simulink library "GRC_Lib"  (R2017b)
settings: Solver=VariableStepAuto  StartTime=0.0  StopTime=10.0  RelTol=1e-3  EnableMultiTasking=on
StartFcn:
  | set_param('AdvancedOperations','ZoomFactor','100');
undefined symbols (not defined in the file): Test
libraries: GRC_Lib x203, simulink x1
(part 2 of 4)

== system GRC_Lib/Constants_Parameters ==
  note: // 1D/2D Lookup Table just allow
      | -- 'double' input data type
      | -- 'Linear' Lookup method
  CalConstant : Subsystem  mask{slddName=CalParam.sldd, CalParamNameMsk=Test, IniVal=0, CPDT=double, MinVal=0, MaxVal=10, StrgClss=SimulinkGlobal}
      mask prompts: slddName "Linked sldd Name"; CalParamNameMsk "Calibration Parameter Name"; IniVal "Initial Value"; CPDT "Calibration Parameter Data Type"; MinVal "Min Value"; MaxVal "Max Value"; StrgClss "Storage Class"
      mask init:
      | CalParamName = CalParamNameMsk;
      | ParamVal = IniVal;
      | ParamMin = MinVal;
      | ParamMax = MaxVal;
      | 
      | set_param(gcb,'slddName',get_param(gcs,'DataDictionary'));
      | % slddName = get_param(gcs,'DataDictionary')
      | 
      | Caldd = Simulink.data.dictionary.open(get_param(gcs,'DataDictionary'));  
      | clc;
      | if ~exist(getSection(Caldd,'Design Data'),get_param(gcb,'CalParamNameMsk'))
      |     importFromFile(getSection(Caldd,'Design Data'),'CalParamDef.m');
      | else
      |     warning('*** The parameter %s has added to sldd, please confirm ***',get_param(gcb,'CalParamNameMsk'));
      | end
      | 
      | try
      | if exist(getSection(Caldd,'Design Data'),'Test')
      |     deleteEntry(getEntry(getSection(Simulink.data.dictionary.open(get_param(gcs,'DataDictionary')),'Design Data'),'Test'));
      | else
      | end
      | catch
      | end
      | 
      | saveChanges(Caldd);
      | fprintf('%s save finished.\n',get_param(gcb,'slddName')); 
      | clear;
      | 
      | DTStry = get_param(gcb,'CPDT');
      | try
      |     if isequal(DTStry,'boolean')
      |         FColor = '[0.901961, 0.313725, 0.078431]'; 
      |     elseif isequal(DTStry,'double')||isequal(DTStry,'single')
      |         FColor = '[0.313725, 0.117647, 0.352941]';  
      |     else
      |         FColor = '[0.196078, 0.549020, 0.549020]';
      |     end        
      | catch
      | end
      | set_param([gcb '/Out'],'ForegroundColor',FColor);
      | set_param(gcb,'ForegroundColor',FColor);
      settings: AttributesFormatString=%<slddName>
      mask Callback CalParamNameMsk:
      | FileFullPath = which(get_param(gcs,'DataDictionary'));
      | [ParentPathStr,name,ext] = fileparts(FileFullPath);
      | cd(ParentPathStr);
      | 
      | if ~exist(getSection(Simulink.data.dictionary.open(get_param(gcs,'DataDictionary')),'Design Data'),get_param(gcb,'CalParamNameMsk'))
      | %    try
      |    fid = fopen('CalParamDef.m','w');
      |    fprintf(fid,'%s',strcat(get_param(gcb,'CalParamNameMsk'),' = Simulink.Parameter;'));
      |    fprintf(fid,'\r');
      |    fprintf(fid,'%s',strcat(get_param(gcb,'CalParamNameMsk'),'.Value = ',get_param(gcb,'IniVal'),';'));
      |    fprintf(fid,'\r');
      |    fprintf(fid,'%s',strcat(get_param(gcb,'CalParamNameMsk'),'.Min = ',get_param(gcb,'MinVal'),';'));
      |    fprintf(fid,'\r');
      |    fprintf(fid,'%s',strcat(get_param(gcb,'CalParamNameMsk'),'.Max = ',get_param(gcb,'MaxVal'),';'));
      |    fprintf(fid,'\r');
      |    fprintf(fid,'%s',strcat(get_param(gcb,'CalParamNameMsk'),'.DataType = ','''', get_param(gcb,'CPDT')),'''',';');
      |    fprintf(fid,'\r');
      |    fprintf(fid,'%s',strcat(get_param(gcb,'CalParamNameMsk'),'.StorageClass = ','''',get_param(gcb,'StrgClss')),'''',';');
      |    fclose(fid);
      | %    catch
      | %    end
      | clear;
      | clc;
      | else
      | end
      mask Callback IniVal:
      | FileFullPath = which(get_param(gcs,'DataDictionary'));
      | [ParentPathStr,name,ext] = fileparts(FileFullPath);
      | cd(ParentPathStr);
      | 
      | if ~exist(getSection(Simulink.data.dictionary.open(get_param(gcs,'DataDictionary')),'Design Data'),get_param(gcb,'CalParamNameMsk'))
      | %    try
      |    fid = fopen('CalParamDef.m','w');
      |    fprintf(fid,'%s',strcat(get_param(gcb,'CalParamNameMsk'),' = Simulink.Parameter;'));
      |    fprintf(fid,'\r');
      |    fprintf(fid,'%s',strcat(get_param(gcb,'CalParamNameMsk'),'.Value = ',get_param(gcb,'IniVal'),';'));
      |    fprintf(fid,'\r');
      |    fprintf(fid,'%s',strcat(get_param(gcb,'CalParamNameMsk'),'.Min = ',get_param(gcb,'MinVal'),';'));
      |    fprintf(fid,'\r');
      |    fprintf(fid,'%s',strcat(get_param(gcb,'CalParamNameMsk'),'.Max = ',get_param(gcb,'MaxVal'),';'));
      |    fprintf(fid,'\r');
      |    fprintf(fid,'%s',strcat(get_param(gcb,'CalParamNameMsk'),'.DataType = ','''', get_param(gcb,'CPDT')),'''',';');
      |    fprintf(fid,'\r');
      |    fprintf(fid,'%s',strcat(get_param(gcb,'CalParamNameMsk'),'.StorageClass = ','''',get_param(gcb,'StrgClss')),'''',';');
      |    fclose(fid);
      | %    catch
      | %    end
      | clear;
      | clc;
      | else
      | end
      mask Callback CPDT:
      | FileFullPath = which(get_param(gcs,'DataDictionary'));
      | [ParentPathStr,name,ext] = fileparts(FileFullPath);
      | cd(ParentPathStr);
      | 
      | if ~exist(getSection(Simulink.data.dictionary.open(get_param(gcs,'DataDictionary')),'Design Data'),get_param(gcb,'CalParamNameMsk'))
      | %    try
      |    fid = fopen('CalParamDef.m','w');
      |    fprintf(fid,'%s',strcat(get_param(gcb,'CalParamNameMsk'),' = Simulink.Parameter;'));
      |    fprintf(fid,'\r');
      |    fprintf(fid,'%s',strcat(get_param(gcb,'CalParamNameMsk'),'.Value = ',get_param(gcb,'IniVal'),';'));
      |    fprintf(fid,'\r');
      |    fprintf(fid,'%s',strcat(get_param(gcb,'CalParamNameMsk'),'.Min = ',get_param(gcb,'MinVal'),';'));
      |    fprintf(fid,'\r');
      |    fprintf(fid,'%s',strcat(get_param(gcb,'CalParamNameMsk'),'.Max = ',get_param(gcb,'MaxVal'),';'));
      |    fprintf(fid,'\r');
      |    fprintf(fid,'%s',strcat(get_param(gcb,'CalParamNameMsk'),'.DataType = ','''', get_param(gcb,'CPDT')),'''',';');
      |    fprintf(fid,'\r');
      |    fprintf(fid,'%s',strcat(get_param(gcb,'CalParamNameMsk'),'.StorageClass = ','''',get_param(gcb,'StrgClss')),'''',';');
      |    fclose(fid);
      | %    catch
      | %    end
      | clear;
      | clc;
      | else
      | end
      mask Callback MinVal:
      | FileFullPath = which(get_param(gcs,'DataDictionary'));
      | [ParentPathStr,name,ext] = fileparts(FileFullPath);
      | cd(ParentPathStr);
      | 
      | if ~exist(getSection(Simulink.data.dictionary.open(get_param(gcs,'DataDictionary')),'Design Data'),get_param(gcb,'CalParamNameMsk'))
      | %    try
      |    fid = fopen('CalParamDef.m','w');
      |    fprintf(fid,'%s',strcat(get_param(gcb,'CalParamNameMsk'),' = Simulink.Parameter;'));
      |    fprintf(fid,'\r');
      |    fprintf(fid,'%s',strcat(get_param(gcb,'CalParamNameMsk'),'.Value = ',get_param(gcb,'IniVal'),';'));
      |    fprintf(fid,'\r');
      |    fprintf(fid,'%s',strcat(get_param(gcb,'CalParamNameMsk'),'.Min = ',get_param(gcb,'MinVal'),';'));
      |    fprintf(fid,'\r');
      |    fprintf(fid,'%s',strcat(get_param(gcb,'CalParamNameMsk'),'.Max = ',get_param(gcb,'MaxVal'),';'));
      |    fprintf(fid,'\r');
      |    fprintf(fid,'%s',strcat(get_param(gcb,'CalParamNameMsk'),'.DataType = ','''', get_param(gcb,'CPDT')),'''',';');
      |    fprintf(fid,'\r');
      |    fprintf(fid,'%s',strcat(get_param(gcb,'CalParamNameMsk'),'.StorageClass = ','''',get_param(gcb,'StrgClss')),'''',';');
      |    fclose(fid);
      | %    catch
      | %    end
      | clear;
      | clc;
      | else
      | end
      mask Callback MaxVal:
      | FileFullPath = which(get_param(gcs,'DataDictionary'));
      | [ParentPathStr,name,ext] = fileparts(FileFullPath);
      | cd(ParentPathStr);
      | 
      | if ~exist(getSection(Simulink.data.dictionary.open(get_param(gcs,'DataDictionary')),'Design Data'),get_param(gcb,'CalParamNameMsk'))
      | %    try
      |    fid = fopen('CalParamDef.m','w');
      |    fprintf(fid,'%s',strcat(get_param(gcb,'CalParamNameMsk'),' = Simulink.Parameter;'));
      |    fprintf(fid,'\r');
      |    fprintf(fid,'%s',strcat(get_param(gcb,'CalParamNameMsk'),'.Value = ',get_param(gcb,'IniVal'),';'));
      |    fprintf(fid,'\r');
      |    fprintf(fid,'%s',strcat(get_param(gcb,'CalParamNameMsk'),'.Min = ',get_param(gcb,'MinVal'),';'));
      |    fprintf(fid,'\r');
      |    fprintf(fid,'%s',strcat(get_param(gcb,'CalParamNameMsk'),'.Max = ',get_param(gcb,'MaxVal'),';'));
      |    fprintf(fid,'\r');
      |    fprintf(fid,'%s',strcat(get_param(gcb,'CalParamNameMsk'),'.DataType = ','''', get_param(gcb,'CPDT')),'''',';');
      |    fprintf(fid,'\r');
      |    fprintf(fid,'%s',strcat(get_param(gcb,'CalParamNameMsk'),'.StorageClass = ','''',get_param(gcb,'StrgClss')),'''',';');
      |    fclose(fid);
      | %    catch
      | %    end
      | clear;
      | clc;
      | else
      | end
      mask TypeOptions StrgClss: SimulinkGlobal | ExportedGlobal | ImportedGlobal | ImportedExternPointer | Default (Custom) | BitField (Custom) | Const (Custom) | Volatile (Custom) | ConstVolatile (Custom) | Define (Custom) | ImportedDefine (Custom) | ExportToFile (Custom) | ImportFromFile (Custom) | FileScope (Custom) | Struct (Custom) | GetSet (Custom) | CompilerFlag (Custom)
      mask Callback StrgClss:
      | FileFullPath = which(get_param(gcs,'DataDictionary'));
      | [ParentPathStr,name,ext] = fileparts(FileFullPath);
      | cd(ParentPathStr);
      | 
      | if ~exist(getSection(Simulink.data.dictionary.open(get_param(gcs,'DataDictionary')),'Design Data'),get_param(gcb,'CalParamNameMsk'))
      | %    try
      |    fid = fopen('CalParamDef.m','w');
      |    fprintf(fid,'%s',strcat(get_param(gcb,'CalParamNameMsk'),' = Simulink.Parameter;'));
      |    fprintf(fid,'\r');
      |    fprintf(fid,'%s',strcat(get_param(gcb,'CalParamNameMsk'),'.Value = ',get_param(gcb,'IniVal'),';'));
      |    fprintf(fid,'\r');
      |    fprintf(fid,'%s',strcat(get_param(gcb,'CalParamNameMsk'),'.Min = ',get_param(gcb,'MinVal'),';'));
      |    fprintf(fid,'\r');
      |    fprintf(fid,'%s',strcat(get_param(gcb,'CalParamNameMsk'),'.Max = ',get_param(gcb,'MaxVal'),';'));
      |    fprintf(fid,'\r');
      |    fprintf(fid,'%s',strcat(get_param(gcb,'CalParamNameMsk'),'.DataType = ','''', get_param(gcb,'CPDT')),'''',';');
      |    fprintf(fid,'\r');
      |    fprintf(fid,'%s',strcat(get_param(gcb,'CalParamNameMsk'),'.StorageClass = ','''',get_param(gcb,'StrgClss')),'''',';');
      |    fclose(fid);
      | %    catch
      | %    end
      | clear;
      | clc;
      | else
      | end
      mask DialogControl Container5 Prompt: sldd link
      mask DialogControl Container6 Prompt: Calibration Parameter
      mask Display:
      | color('black');
      | disp(get_param(gcb,'CalParamNameMsk'));
  Stdrd1DLookupTable : Subsystem  TreatAsAtomicUnit=on  mask{method=Linear, Tbl_U_Name=[-pi:pi/50:pi], Tbl_y_Name=sin([-pi:pi/50:pi]), OpDT=double}
      mask prompts: method "Lookup method"; Tbl_U_Name "Vector of input values"; Tbl_y_Name "Table data"; OpDT "Output Data Type"
      mask init:
      | MethodStr = get_param(gcb,'method');
      | UStr = get_param(gcb,'Tbl_U_Name');
      | yStr = get_param(gcb,'Tbl_y_Name');
      | DTStr = get_param(gcb,'OpDT');
      | %if isequal(MethodStr,'Linear')
      |     try
      |     set_param([gcb '/Stdrd1DTable'],'InterpMethod',MethodStr);
      |     set_param([gcb '/Stdrd1DTable'],'BreakpointsForDimension1',UStr);
      |     set_param([gcb '/Stdrd1DTable'],'Table',yStr);
      |     
      |     set_param([gcb '/Stdrd1DTable'],'TableDataTypeStr',DTStr);
      |     set_param([gcb '/Stdrd1DTable'],'IntermediateResultsDataTypeStr',DTStr);
      |     set_param([gcb '/Stdrd1DTable'],'FractionDataTypeStr',DTStr);
      |     set_param([gcb '/Stdrd1DTable'],'OutDataTypeStr',DTStr);
      |     set_param([gcb '/Stdrd1DTable'],'BreakpointsForDimension1DataTypeStr',DTStr); 
      |     catch
      |     end
      |     
      | 
      | FColor = '[0.313725, 0.117647, 0.352941]'; 
      | try
      |     set_param([gcb '/y'],'ForegroundColor',FColor);
      |     set_param(gcb,'ForegroundColor',FColor);
      | catch
      | end
      settings: AttributesFormatString=%<OpDT>
      mask TypeOptions method: Flat | Nearest | Linear | Cubic spline
      mask Display:
      | color('blue')
      | plot(Tbl_U_Name,Tbl_y_Name);
  Stdrd2DLookupTable : Subsystem  TreatAsAtomicUnit=on  mask{method=Linear, Tbl_BP1_Name=[1 2 3 4], Tbl_BP2_Name=[1 2 3], Tbl_Tbl_Name=[4 5 6;15 17 19;10 15 23;5 13 20], OpDT=double}
      mask prompts: method "Lookup method"; Tbl_BP1_Name "Vector of breakpoints 1"; Tbl_BP2_Name "Vector of breakpoints 2"; Tbl_Tbl_Name "Table data"; OpDT "Output Data Type"
      mask init:
      | MethodStr = get_param(gcb,'method');
      | BP1Str = get_param(gcb,'Tbl_BP1_Name');
      | BP2Str = get_param(gcb,'Tbl_BP2_Name');
      | TblStr = get_param(gcb,'Tbl_Tbl_Name');
      | DTStr = get_param(gcb,'OpDT');
      | 
      | try
      | set_param([gcb '/Stdrd2DTable'],'InterpMethod',MethodStr);
      | set_param([gcb '/Stdrd2DTable'],'BreakpointsForDimension1',BP1Str);
      | set_param([gcb '/Stdrd2DTable'],'BreakpointsForDimension2',BP2Str);
      | set_param([gcb '/Stdrd2DTable'],'Table',TblStr);
      | 
      | set_param([gcb '/Stdrd2DTable'],'TableDataTypeStr',DTStr);
      | set_param([gcb '/Stdrd2DTable'],'IntermediateResultsDataTypeStr',DTStr);
      | set_param([gcb '/Stdrd2DTable'],'FractionDataTypeStr',DTStr);
      | set_param([gcb '/Stdrd2DTable'],'OutDataTypeStr',DTStr);
      | set_param([gcb '/Stdrd2DTable'],'BreakpointsForDimension1DataTypeStr',DTStr); 
      | set_param([gcb '/Stdrd2DTable'],'BreakpointsForDimension2DataTypeStr',DTStr); 
      | catch
      | end
      | 
      | FColor = '[0.313725, 0.117647, 0.352941]'; 
      | try
      |     set_param([gcb '/out'],'ForegroundColor',FColor);
      |     set_param(gcb,'ForegroundColor',FColor);
      | catch
      | end
      settings: AttributesFormatString=%<OpDT>
      mask TypeOptions method: Flat | Nearest | Linear | Cubic spline
      mask Display:
      | % x = [1 2 3];
      | % y1 = [4 15 10];
      | % y2 = [5 17 15];
      | % y3 = [6 19 23];
      | % color('blue');
      | % plot(x,y1,x,y2,x,y3);
      | 
      | color('blue')
      | for i = 1 : length(Tbl_BP2_Name)
      |     plot(Tbl_BP1_Name,Tbl_Tbl_Name(:,i));
      |     hold on;
      | end
      | close(gcf);

== system GRC_Lib/Counter_Timer ==
  RstCntDwn : Subsystem  TreatAsAtomicUnit=on  mask{IpDT=uint16}
      mask prompts: IpDT "Input RstV Data Type"
      mask init:
      | DTStr = get_param(gcb,'IpDT');
      | set_param([gcb '/Constant'],'OutDataTypeStr',DTStr); 
      | set_param([gcb '/Constant1'],'OutDataTypeStr',DTStr); 
      | set_param([gcb '/SUB_Uint'],'IpDT',DTStr); 
      | 
      | FColor = '[0.901961, 0.313725, 0.078431]'; 
      | try
      |     set_param([gcb '/y'],'ForegroundColor',FColor);
      |     set_param(gcb,'ForegroundColor',FColor);
      | catch
      | end
      mask Display:
      | % color('red');
      | % disp ('RstCntDwn\n(8|16|32bit)');
      | image(imread('RstCntDwn.jpg'),[0.2,0.1,0.7,0.85]);
  RstCntStpRise : Subsystem  TreatAsAtomicUnit=on  mask{IpDT=uint8}
      mask prompts: IpDT "Input RstV Data Type"
      mask init:
      | DTStr = get_param(gcb,'IpDT');
      | set_param([gcb '/Constant'],'OutDataTypeStr',DTStr); 
      | set_param([gcb '/SUM'],'IpDT',DTStr); 
      | 
      | DTStry = get_param([gcb '/Constant'],'OutDataTypeStr');
      | try
      |     if isequal(DTStry,'boolean')
      |         FColor = '[0.901961, 0.313725, 0.078431]'; 
      |     elseif isequal(DTStry,'double')||isequal(DTStry,'single')
      |         FColor = '[0.313725, 0.117647, 0.352941]';  
      |     else
      |         FColor = '[0.196078, 0.549020, 0.549020]';
      |     end        
      | catch
      | end
      | set_param([gcb '/Cntr'],'ForegroundColor',FColor);
      | set_param(gcb,'ForegroundColor',FColor);
      mask Display:
      | % color('blue');
      | % disp ('RstCntStpRise\n(8|16|32bit)');
      | image(imread('RstCntStpRise.jpg'),[0.2,0.05,0.6,0.9]);
  RstTmr : Subsystem  TreatAsAtomicUnit=on  mask{IpDT=double}
      mask prompts: IpDT "Input Data Type (RstV and dT)"
      mask help:
      | %%% Output Tmr
      | if   (RstV<dT*0.5)
      |  	 Tmr = 0;
      | elseif  (Rst)
      | 	 Tmr = RstV+dT*0.5;
      | elseif  (E && Tmr(-1)>0)
      |  	 Tmr = Tmr(-1) - dT;
      | else
      |   	 Tmr = Tmr(-1);
      | %%% Output y
      | if  (out > 0)
      | 	  y = boolean(1);
      | else
      |   	 y = boolean(0);
      mask init:
      | DTStr = get_param(gcb,'IpDT');
      | set_param([gcb '/Constant'],'OutDataTypeStr',DTStr); 
      | set_param([gcb '/Constant1'],'OutDataTypeStr',DTStr); 
      | set_param([gcb '/Constant2'],'OutDataTypeStr',DTStr); 
      | set_param([gcb '/GAIN'],'IpDT',DTStr); 
      | set_param([gcb '/SUM'],'IpDT',DTStr); 
      | set_param([gcb '/SUB'],'IpDT',DTStr); 
      | 
      | FColor = '[0.901961, 0.313725, 0.078431]'; 
      | try
      |     set_param([gcb '/y'],'ForegroundColor',FColor);
      |     set_param(gcb,'ForegroundColor',FColor);
      | catch
      | end
      mask Display:
      | % color('blue');
      | % disp ('RstTmr');
      | image(imread('RstTmr.jpg'),[0.2,0.1,0.7,0.85]);
  RstTmrZero : Subsystem  TreatAsAtomicUnit=on  mask{IpDT=double}
      mask prompts: IpDT "Input Data Type (RstV and dT)"
      mask help:
      | %%% Output Tmr
      | if   (RstV<dT*0.5)
      |  	 Tmr = 0;
      | elseif  (Rst && Tmr(-1)<=0)
      | 	 Tmr = RstV+dT*0.5;
      | elseif  (E && Tmr(-1)>0)
      |  	 Tmr = Tmr(-1) - dT;
      | else
      |   	 Tmr = Tmr(-1);
      | %%% Output y
      | if  (out > 0)
      | 	  y = boolean(1);
      | else
      |   	 y = boolean(0);
      mask init: same as GRC_Lib/Counter_Timer/RstTmr
      mask Display:
      | % color('blue');
      | % disp ('RstTmrZero');
      | image(imread('RstTmrZero.jpg'),[0.2,0.1,0.7,0.85]);
  StopWatch : Subsystem  TreatAsAtomicUnit=on  mask{IpDT=single}
      mask prompts: IpDT "Input dT Data Type"
      mask init:
      | DTStr = get_param(gcb,'IpDT');
      | set_param([gcb '/Constant'],'OutDataTypeStr',DTStr); 
      | set_param([gcb '/SUM'],'IpDT',DTStr); 
      | 
      | DTStry = get_param([gcb '/Constant'],'OutDataTypeStr');
      | try
      |     if isequal(DTStry,'boolean')
      |         FColor = '[0.901961, 0.313725, 0.078431]'; 
      |     elseif isequal(DTStry,'double')||isequal(DTStry,'single')
      |         FColor = '[0.313725, 0.117647, 0.352941]';  
      |     else
      |         FColor = '[0.196078, 0.549020, 0.549020]';
      |     end        
      | catch
      | end
      | set_param([gcb '/Tmr'],'ForegroundColor',FColor);
      | set_param(gcb,'ForegroundColor',FColor);
      mask Display:
      | % color('blue');
      | % disp ('StopWatch');
      | image(imread('StopWatch.jpg'),[0.2,0.05,0.6,0.9]);

== system GRC_Lib/Delay ==
  Delay : Subsystem  TreatAsAtomicUnit=on  mask{IniV=0, IpDT=double}
      mask prompts: IniV "Initial Value"; IpDT "Input Data Type"
      mask init:
      | IniStr = get_param(gcb,'IniV');
      | try
      |     set_param([gcb '/UnitDelay'],'InitialCondition',IniStr);
      | catch
      | end
      mask Display:
      | color('green');
      | dpoly([0,1],[1,0],'z');
  DelayIniV : Subsystem  TreatAsAtomicUnit=on
      mask help: Unit delay, while the initial value is input from port1 and the input u can't be vector.
      mask Display:
      | color('green');
      | dpoly([0,1],[1,0],'z');
  InitStp : Subsystem  TreatAsAtomicUnit=on  mask{OpDT_B=on, StpTp=~0 to 0, InitV=5, FnlV=5}
      mask prompts: OpDT_B "Output Boolean"; StpTp "Step Type"; InitV "Initial Value"; FnlV "Final Value"
      mask init:
      | %%% Input parameter detection
      | try
      |     DTBStr =  get_param(gcb,'OpDT_B');    
      |     if isequal(DTBStr,'on')      
      |       set_param(gcb,'MaskEnableString','on,on,off,off');
      |       set_param(gcb,'MaskVisibilityString','on,on,off,off');
      |       StpTpStr =  get_param(gcb,'StpTp');          
      |         if strcmp(get_param(gcb,'StpTp'),'~0 to 0')
      |            set_param(gcb,'MaskEnableString','on,on,on,off');
      |            set_param(gcb,'MaskVisibilityString','on,on,on,off'); 
      |            set_param([gcb '/Cnst'],'Value','0');
      |            set_param([gcb '/Cnst'],'OutDataTypeStr','boolean');
      |            set_param([gcb '/Delay'],'InitialCondition','1');
      |         else
      |            set_param(gcb,'MaskEnableString','on,on,off,on');
      |            set_param(gcb,'MaskVisibilityString','on,on,off,on'); 
      |            set_param([gcb '/Cnst'],'Value','1');
      |            set_param([gcb '/Cnst'],'OutDataTypeStr','boolean');
      |            set_param([gcb '/Delay'],'InitialCondition','0');
      |         end
      |     else
      |       set_param(gcb,'MaskEnableString','on,on,on,on');
      |       set_param(gcb,'MaskVisibilityString','on,on,on,on');
      |       StpTpStr =  get_param(gcb,'StpTp');
      |         if strcmp(get_param(gcb,'StpTp'),'~0 to 0')
      |             set_param(gcb,'MaskEnableString','on,on,on,off');
      |             set_param(gcb,'MaskVisibilityString','on,on,on,off'); 
      |             set_param([gcb '/Cnst'],'Value','0');
      |             set_param([gcb '/Cnst'],'OutDataTypeStr','double');
      |             set_param([gcb '/Delay'],'InitialCondition',get_param(gcbh,'InitV'));      
      |         else
      |             set_param(gcb,'MaskEnableString','on,on,off,on');
      |             set_param(gcb,'MaskVisibilityString','on,on,off,on'); 
      |             set_param([gcb '/Cnst'],'Value',get_param(gcbh,'FnlV'));
      |             set_param([gcb '/Cnst'],'OutDataTypeStr','double');
      |             set_param([gcb '/Delay'],'InitialCondition','0');
      |         end
      |     end
      | catch
      | end
      | 
      | DTStry = get_param([gcb '/Cnst'],'OutDataTypeStr');
      | try
      |     if isequal(DTBStr,'on')
      |         FColor = '[0.901961, 0.313725, 0.078431]'; 
      |     elseif isequal(DTBStr,'off') && isequal(DTStry,'double')
      |         FColor = '[0.313725, 0.117647, 0.352941]';  
      |     else
      |     end        
      | catch
      | end
      | set_param([gcb '/y'],'ForegroundColor',FColor);
      | set_param(gcb,'ForegroundColor',FColor);
      mask Callback OpDT_B:
      | if isequal(get_param(gcb,'OpDT_B'),'on')
      |    set_param(gcb,'MaskEnableString','on,on,off,off');
      |    set_param(gcb,'MaskVisibilityString','on,on,off,off');
      | else
      |    set_param(gcb,'MaskEnableString','on,on,on,on');
      |    set_param(gcb,'MaskVisibilityString','on,on,on,on');
      | end
      mask TypeOptions StpTp: 0 to ~0 | ~0 to 0
      mask Callback StpTp:
      | if strcmp(get_param(gcb,'StpTp'),'~0 to 0')
      |    set_param(gcb,'MaskEnableString','on,on,on,off');
      |    set_param(gcb,'MaskVisibilityString','on,on,on,off');
      | else
      |    set_param(gcb,'MaskEnableString','on,on,off,on');
      |    set_param(gcb,'MaskVisibilityString','on,on,off,on');
      | end
      mask Display:
      | color('green');
      | plot([0.25 0.7],double([1 1]));
      | plot([0.2 0.25],double([0 0]));
      | plot([0.25 0.25],[1 0]);
  TurnOffDelay : Subsystem  TreatAsAtomicUnit=on  mask{IpDT=double}
      mask prompts: IpDT "Input Data Type (T and dT)"
      mask init:
      | DTStr = get_param(gcb,'IpDT');
      | 
      | set_param([gcb '/GAIN'],'IpDT',DTStr);
      | set_param([gcb '/SUB1'],'IpDT',DTStr);
      | set_param([gcb '/SUB2'],'IpDT',DTStr);
      | set_param([gcb '/Constant'],'OutDataTypeStr',DTStr);
      | set_param([gcb '/Constant1'],'OutDataTypeStr',DTStr);
      | 
      | FColor = '[0.901961, 0.313725, 0.078431]'; 
      | try
      |     set_param([gcb '/y'],'ForegroundColor',FColor);
      |     set_param(gcb,'ForegroundColor',FColor);
      | catch
      | end
      mask Display:
      | % color('red');
      | % disp (sprintf('Delay\n(TurnOff ↓)'));
      | image(imread('TurnOffDelay.jpg'),[0.25,0.1,0.6,0.8]);
  TurnOffDelay_Dyn : Subsystem  TreatAsAtomicUnit=on  mask{IpDT=double}
      mask prompts: IpDT "Input Data Type (T and dT)"
      mask init:
      | DTStr = get_param(gcb,'IpDT');
      | 
      | set_param([gcb '/GAIN'],'IpDT',DTStr);
      | set_param([gcb '/SUM'],'IpDT',DTStr);
      | set_param([gcb '/SUB'],'IpDT',DTStr);
      | set_param([gcb '/Constant1'],'OutDataTypeStr',DTStr);
      | set_param([gcb '/Constant2'],'OutDataTypeStr',DTStr);
      | 
      | FColor = '[0.901961, 0.313725, 0.078431]'; 
      | try
      |     set_param([gcb '/y'],'ForegroundColor',FColor);
      |     set_param(gcb,'ForegroundColor',FColor);
      | catch
      | end
      mask Display: image(imread('TurnOffDelay_Dyn.jpg'),[0.25,0.1,0.6,0.8]);
  TurnOnDelay : Subsystem  TreatAsAtomicUnit=on  mask{IpDT=double}
      mask prompts: IpDT "Input Data Type (T and dT)"
      mask init: same as GRC_Lib/Delay/TurnOffDelay
      mask Display:
      | % color('red');
      | % disp (sprintf('Delay\n(TurnOn ↑)'));
      | image(imread('TurnOnDelay.jpg'),[0.25,0.1,0.6,0.8]);
  TurnOnDelay_Dyn : Subsystem  TreatAsAtomicUnit=on  mask{IpDT=single}
      mask prompts: IpDT "Input Data Type (T and dT)"
      mask init: same as GRC_Lib/Delay/TurnOffDelay_Dyn
      mask Display: image(imread('TurnOnDelay_Dyn.jpg'),[0.25,0.1,0.6,0.8]);

== system GRC_Lib/Extras ==

== system GRC_Lib/Filter ==
  DigitalLowPass : Subsystem  TreatAsAtomicUnit=on  mask{IpDT=single}
      mask prompts: IpDT "Input Data Type (RstV, m and u)"
      mask init:
      | DTStr = get_param(gcb,'IpDT');
      | 
      | set_param([gcb '/SUB'],'IpDT',DTStr);
      | set_param([gcb '/MUL'],'IpDT',DTStr);
      | set_param([gcb '/SUM'],'IpDT',DTStr);
      | 
      | DTStry = get_param([gcb '/SUM'],'IpDT');
      | try
      |     if isequal(DTStry,'boolean')
      |         FColor = '[0.901961, 0.313725, 0.078431]'; 
      |     elseif isequal(DTStry,'double')||isequal(DTStry,'single')
      |         FColor = '[0.313725, 0.117647, 0.352941]';  
      |     else
      |         FColor = '[0.196078, 0.549020, 0.549020]';
      |     end        
      | catch
      | end
      | set_param([gcb '/y'],'ForegroundColor',FColor);
      | set_param(gcb,'ForegroundColor',FColor);
      mask Display:
      | % color('red');
      | % disp (sprintf('Filter\n(LowPass)'));
      | image(imread('DigitalLowPass.jpg'),[0.3,0.1,0.6,0.8]);
  LowPass_NoTrigger : Subsystem  mask{IpDT=double}
      mask prompts: IpDT "Input Data Type (m and u)"
      mask init: same as GRC_Lib/Filter/DigitalLowPass
      mask Display: image(imread('DigitalLowPass.jpg'),[0.3,0.1,0.6,0.8]);

== system GRC_Lib/Governor ==

== system GRC_Lib/Intergrator ==
  Accumulator : Subsystem  TreatAsAtomicUnit=on  mask{IpDT=int16}
      mask prompts: IpDT "Input Data Type (RstV, u, Min and Max)"
      mask init:
      | DTStr=get_param(gcb,'IpDT');
      | set_param([gcb '/SUM'],'IpDT',DTStr);
      | 
      | DTStry = get_param([gcb '/SUM'],'IpDT');
      | try
      |     if isequal(DTStry,'boolean')
      |         FColor = '[0.901961, 0.313725, 0.078431]'; 
      |     elseif isequal(DTStry,'double')||isequal(DTStry,'single')
      |         FColor = '[0.313725, 0.117647, 0.352941]';  
      |     else
      |         FColor = '[0.196078, 0.549020, 0.549020]';
      |     end        
      | catch
      | end
      | set_param([gcb '/y'],'ForegroundColor',FColor);
      | set_param(gcb,'ForegroundColor',FColor);
      mask Display:
      | % color('red');
      | % disp('\bf∑','texmode','on');
      | image(imread('Accumulator.jpg'),[0.3,0.25,0.3,0.5]);

== system GRC_Lib/LogicalOperation ==
  AND : Subsystem  mask{n=2}
      mask prompts: n "Number of input ports (Min 2)"
      mask init:
      | %%% Input port number detection 
      | if isequal(str2num(get_param(gcb,'n')),[])
      |     if n<2
      |         error('*** ERROR_11 ***    Number of Input Port must be an Integer and >2.');
      |     else
      |     end
      | else
      |     nLgth = str2num(get_param(gcb,'n'));
      |     if nLgth<2
      |         error('*** ERROR_21 ***    Number of Input Port must be an Integer and >2.');
      |     else
      |     end
      | end
      | 
      | LocVal = get_param(gcb,'n');
      | 
      | try
      |     IpNmbr = length(get_param(gcb,'Blocks'))-2;
      |     if str2num(LocVal)<IpNmbr
      |        for j = (str2num(LocVal)+1):IpNmbr
      |             delete_line(gcb, ['In' int2str(j) '/1'], ['AND1/' int2str(j)]);
      |             dlte_block = strcat(gcb,'/',['In' int2str(j)]);
      |             delete_block(dlte_block);  %%% Delete existing Input lines
      |        end
      |        set_param([gcb '/AND1'],'Inputs',LocVal);
      |     elseif str2num(LocVal)>IpNmbr
      |         set_param([gcb '/AND1'],'Inputs',LocVal);    
      |         for i = (IpNmbr+1) : str2num(LocVal)
      |             add_block('simulink/Sources/In1',[gcb '/In' int2str(i)]); %%% Add blocks again
      |             set_param([gcb '/In' int2str(i)],'Position',[-45 13+60*(i-1) -15 27+60*(i-1)]);
      |             add_line(gcb,['In' int2str(i) '/1'],['AND1/' int2str(i)]);       
      |         end  
      |     else
      |         set_param([gcb '/AND1'],'Inputs',LocVal); 
      |     end
      | catch
      | end
      | 
      | FColor = '[0.901961, 0.313725, 0.078431]'; 
      | try
      |     set_param([gcb '/Out'],'ForegroundColor',FColor);
      |     set_param(gcb,'ForegroundColor',FColor);
      | catch
      | end
      mask Callback n:
      | % %%% Input port number detection
      | if isequal(str2num(get_param(gcb,'n')),[])
      |    error('*** ERROR_1 ***    Number of Input Port can not be a %s.',class(get_param(gcb,'n')));
      | elseif str2num(get_param(gcb,'n'))<2
      |    error('*** ERROR_2 ***    Number of Input Port must be an Integer and >2.');
      | else
      | end
      mask Display:
      | color('green');
      | disp('\bfAND','texmode','on');
  NOT : Subsystem
      mask init:
      | set_param([gcb '/NOT1'],'Operator','NOT');
      | % set_param([gcb '/Out'],'OutDataTypeStr','boolean');
      | 
      | FColor = '[0.901961, 0.313725, 0.078431]'; 
      | try
      |     set_param([gcb '/Out'],'ForegroundColor',FColor);
      |     set_param(gcb,'ForegroundColor',FColor);
      | catch
      | end
      mask Display:
      | color('green');
      | disp('\bfNOT','texmode','on');
  OR : Subsystem  mask{n=2}
      mask prompts: n "Number of input ports (Min 2)"
      mask init:
      | %%% Input port number detection 
      | if isequal(str2num(get_param(gcb,'n')),[])
      |     if n<2
      |         error('*** ERROR_11 ***    Number of Input Port must be an Integer and >2.');
      |     else
      |     end
      | else
      |     nLgth = str2num(get_param(gcb,'n'));
      |     if nLgth<2
      |         error('*** ERROR_21 ***    Number of Input Port must be an Integer and >2.');
      |     else
      |     end
      | end
      | 
      | LocVal = get_param(gcb,'n');
      | 
      | try
      |     IpNmbr = length(get_param(gcb,'Blocks'))-2;
      |     if str2num(LocVal)<IpNmbr
      |        for j = (str2num(LocVal)+1):IpNmbr
      |            delete_line(gcb, ['In' int2str(j) '/1'], ['OR1/' int2str(j)]);
      |            dlte_block = strcat(gcb,'/',['In' int2str(j)]);
      |            delete_block(dlte_block);  %%% Delete existing Input lines
      |        end
      |        set_param([gcb '/OR1'],'Inputs',LocVal);
      |     elseif str2num(LocVal)>IpNmbr
      |         set_param([gcb '/OR1'],'Inputs',LocVal);    
      |         for i = (IpNmbr+1) : str2num(LocVal)
      |             add_block('simulink/Sources/In1',[gcb '/In' int2str(i)]); %%% Add blocks 
      |             set_param([gcb '/In' int2str(i)],'Position',[-45 13+60*(i-1) -15 27+60*(i-1)]);
      |             add_line(gcb,['In' int2str(i) '/1'],['OR1/' int2str(i)]);       
      |         end  
      |     else
      |         set_param([gcb '/OR1'],'Inputs',LocVal); 
      |     end
      | catch
      | end
      | 
      | FColor = '[0.901961, 0.313725, 0.078431]'; 
      | try
      |     set_param([gcb '/Out'],'ForegroundColor',FColor);
      |     set_param(gcb,'ForegroundColor',FColor);
      | catch
      | end
      mask Callback n:
      | % %%% Input port number detection
      | if isequal(str2num(get_param(gcb,'n')),[])
      |    error('*** ERROR_1 ***    Number of Input Port can not be a %s.',class(get_param(gcb,'n')));
      | elseif str2num(get_param(gcb,'n'))<2
      |    error('*** ERROR_2 ***    Number of Input Port must be an Integer and >2.');
      | else
      | end
      mask Display:
      | color('green');
      | disp('\bfOR','texmode','on');
  XOR : Subsystem  mask{n=2}
      mask prompts: n "Number of input ports (Min 2)"
      mask init:
      | %%% Input port number detection 
      | if isequal(str2num(get_param(gcb,'n')),[])
      |     if n<2
      |         error('*** ERROR_11 ***    Number of Input Port must be an Integer and >2.');
      |     else
      |     end
      | else
      |     nLgth = str2num(get_param(gcb,'n'));
      |     if nLgth<2
      |         error('*** ERROR_21 ***    Number of Input Port must be an Integer and >2.');
      |     else
      |     end
      | end
      | 
      | LocVal = get_param(gcb,'n');
      | 
      | try
      |     IpNmbr = length(get_param(gcb,'Blocks'))-2;
      |     if str2num(LocVal)<IpNmbr
      |        for j = (str2num(LocVal)+1):IpNmbr
      |            delete_line(gcb, ['In' int2str(j) '/1'], ['XOR1/' int2str(j)]);
      |            dlte_block = strcat(gcb,'/',['In' int2str(j)]);
      |            delete_block(dlte_block);  %%% Delete existing Input lines
      |        end
      |        set_param([gcb '/XOR1'],'Inputs',LocVal);
      |     elseif str2num(LocVal)>IpNmbr
      |         set_param([gcb '/XOR1'],'Inputs',LocVal);    
      |         for i = (IpNmbr+1) : str2num(LocVal)
      |             add_block('simulink/Sources/In1',[gcb '/In' int2str(i)]); %%% Add blocks 
      |             set_param([gcb '/In' int2str(i)],'Position',[-45 13+60*(i-1) -15 27+60*(i-1)]);
      |             add_line(gcb,['In' int2str(i) '/1'],['XOR1/' int2str(i)]);       
      |         end  
      |     else
      |         set_param([gcb '/XOR1'],'Inputs',LocVal); 
      |     end
      | catch
      | end
      | 
      | FColor = '[0.901961, 0.313725, 0.078431]'; 
      | try
      |     set_param([gcb '/Out'],'ForegroundColor',FColor);
      |     set_param(gcb,'ForegroundColor',FColor);
      | catch
      | end
      mask Callback n:
      | % %%% Input port number detection
      | if isequal(str2num(get_param(gcb,'n')),[])
      |    error('*** ERROR_1 ***    Number of Input Port can not be a %s.',class(get_param(gcb,'n')));
      | elseif str2num(get_param(gcb,'n'))<2
      |    error('*** ERROR_2 ***    Number of Input Port must be an Integer and >2.');
      | else
      | end
      mask Display:
      | color('green');
      | disp('\bfXOR','texmode','on');

== system GRC_Lib/MathFunction ==
  Sqr : Subsystem  TreatAsAtomicUnit=on  mask{IpDT=uint32}
      mask prompts: IpDT "Input Data Type"
      mask init:
      | DTStr = get_param(gcb,'IpDT');
      | try
      |     if isequal(DTStr,'int8')||isequal(DTStr,'uint8')
      |         set_param([gcb '/Square'],'OutDataTypeStr','uint16'); 
      |         %set_param([gcb '/y'],'OutDataTypeStr','uint16');
      |     elseif isequal(DTStr,'int16')||isequal(DTStr,'uint16')
      |         set_param([gcb '/Square'],'OutDataTypeStr','uint32'); 
      |         %set_param([gcb '/y'],'OutDataTypeStr','uint32'); 
      |     elseif isequal(DTStr,'int32')||isequal(DTStr,'uint32')
      |         set_param([gcb '/Square'],'OutDataTypeStr','uint32'); 
      |         %set_param([gcb '/y'],'OutDataTypeStr','uint32'); 
      |     elseif isequal(DTStr,'double')||isequal(DTStr,'single')
      |         set_param([gcb '/Square'],'OutDataTypeStr','double'); 
      |         %set_param([gcb '/y'],'OutDataTypeStr','double'); 
      |     end        
      | catch
      | end
      | 
      | DTStry = get_param([gcb '/Square'],'OutDataTypeStr');
      | try
      |     if isequal(DTStry,'boolean')
      |         FColor = '[0.901961, 0.313725, 0.078431]'; 
      |     elseif isequal(DTStry,'double')||isequal(DTStry,'single')
      |         FColor = '[0.313725, 0.117647, 0.352941]';  
      |     else
      |         FColor = '[0.196078, 0.549020, 0.549020]';
      |     end        
      | catch
      | end
      | set_param([gcb '/y'],'ForegroundColor',FColor);
      | set_param(gcb,'ForegroundColor',FColor);
      mask Display:
      | color('green');
      | disp('\bfu^2','texmode','on');
  Sqrt : Subsystem  TreatAsAtomicUnit=on  mask{Fcn=sqrt, OpDT=double}
      mask prompts: Fcn "Function"; OpDT "Output Data Type"
      mask init:
      | FcnStr = get_param(gcb,'Fcn');
      | set_param([gcb '/Sqrt'],'Operator',FcnStr); 
      | DTStr = get_param(gcb,'OpDT');
      | set_param([gcb '/Sqrt'],'OutDataTypeStr',DTStr); 
      | %set_param([gcb '/y'],'OutDataTypeStr',DTStr); 
      | 
      | DTStry = get_param([gcb '/Sqrt'],'OutDataTypeStr');
      | try
      |     if isequal(DTStry,'boolean')
      |         FColor = '[0.901961, 0.313725, 0.078431]'; 
      |     elseif isequal(DTStry,'double')||isequal(DTStry,'single')
      |         FColor = '[0.313725, 0.117647, 0.352941]';  
      |     else
      |         FColor = '[0.196078, 0.549020, 0.549020]';
      |     end        
      | catch
      | end
      | set_param([gcb '/y'],'ForegroundColor',FColor);
      | set_param(gcb,'ForegroundColor',FColor);
      mask TypeOptions Fcn: sqrt | signedSqrt | rSqrt
      mask Display:
      | color('green');
      | disp('u^-2');

== system GRC_Lib/Memory ==
  ER_FF : Subsystem  TreatAsAtomicUnit=on  mask{FalseVal=0, TrueVal=1}
      mask prompts: FalseVal "False Value"; TrueVal "True Value"
      mask init:
      | falseVal = FalseVal;
      | trueVal = TrueVal;
      | 
      | FColor = '[0.901961, 0.313725, 0.078431]'; 
      | try
      |     set_param([gcb '/y'],'ForegroundColor',FColor);
      |     set_param([gcb '/~y'],'ForegroundColor',FColor);
      |     set_param(gcb,'ForegroundColor',FColor);
      | catch
      | end
      mask Display:
      | color('green');
      | disp (sprintf('FlipFlop\n(ER)'));
  Falling : Subsystem  TreatAsAtomicUnit=on  mask{IniVal=0}
      mask prompts: IniVal "Initial Value"
      mask init:
      | IniStr = get_param(gcb,'IniVal');
      | try
      |     set_param([gcb '/Delay'],'IniV',IniStr);
      | catch
      | end
      | 
      | FColor = '[0.901961, 0.313725, 0.078431]'; 
      | try
      |     set_param([gcb '/Out1'],'ForegroundColor',FColor);
      |     set_param(gcb,'ForegroundColor',FColor);
      | catch
      | end
      mask Display:
      | % color('red');
      | % disp ('Trigger\n(↓)');
      | image(imread('Falling.jpg'),[0.2,0.2,0.6,0.6]);
  RE_FF : Subsystem  TreatAsAtomicUnit=on  mask{FalseVal=0, TrueVal=1}
      mask prompts: FalseVal "False Value"; TrueVal "True Value"
      mask init: same as GRC_Lib/Memory/ER_FF
      mask Display:
      | color('green');
      | disp (sprintf('FlipFlop\n(RE)'));
  Rising : Subsystem  TreatAsAtomicUnit=on  mask{IniVal=0}
      mask prompts: IniVal "Initial Value"
      mask init: same as GRC_Lib/Memory/Falling
      mask Display:
      | % color('red');
      | % disp ('Trigger\n(↑)');
      | image(imread('Rising.jpg'),[0.2,0.2,0.6,0.6]);
  RisingFaling : Subsystem  TreatAsAtomicUnit=on  mask{IniVal=0}
      mask prompts: IniVal "Initial Value"
      mask init: same as GRC_Lib/Memory/Falling
      mask Display:
      | % color('red');
      | % disp ('Trigger\n(↑||↓)');
      | image(imread('RisingFaling.jpg'),[0.2,0.2,0.6,0.6]);

== system GRC_Lib/ModelInfo ==

== system GRC_Lib/Nonlinear ==
  ABS : Subsystem  TreatAsAtomicUnit=on  mask{IpDT=int16}
      mask prompts: IpDT "Input Data Type"
      mask init:
      | try
      | set_param([gcb '/Constant'],'OutDataTypeStr',IpDT);
      | set_param([gcb '/Constant1'],'OutDataTypeStr',IpDT);
      | set_param([gcb '/Product'],'OutDataTypeStr',IpDT);
      | catch
      | end
      | 
      | DTStry = get_param([gcb '/Constant'],'OutDataTypeStr');
      | try
      |     if isequal(DTStry,'boolean')
      |         FColor = '[0.901961, 0.313725, 0.078431]'; 
      |     elseif isequal(DTStry,'double')||isequal(DTStry,'single')
      |         FColor = '[0.313725, 0.117647, 0.352941]';  
      |     else
      |         FColor = '[0.196078, 0.549020, 0.549020]';
      |     end        
      | catch
      | end
      | set_param([gcb '/y'],'ForegroundColor',FColor);
      | set_param(gcb,'ForegroundColor',FColor);
      mask Display:
      | color('green');
      | disp('\bf|u|','texmode','on');
  HysLDlt : Subsystem  TreatAsAtomicUnit=on  mask{IpDT=single}
      mask prompts: IpDT "Input Data Type (R, D and u)"
      mask init:
      | DTStr=get_param(gcb,'IpDT');
      | set_param([gcb '/SUM'],'IpDT',DTStr);
      | 
      | FColor = '[0.901961, 0.313725, 0.078431]'; 
      | try
      |     set_param([gcb '/y'],'ForegroundColor',FColor);
      |     set_param(gcb,'ForegroundColor',FColor);
      | catch
      | end
      mask Display:
      | % color('red');
      | % disp (sprintf('Hysterisis\nL-Dlt'));
      | image(imread('HysLDlt.jpg'),[0.2,0.1,0.65,0.9]);
  HysRDlt : Subsystem  TreatAsAtomicUnit=on  mask{IpDT=double}
      mask prompts: IpDT "Input Data Type (R, D and u)"
      mask init:
      | DTStr=get_param(gcb,'IpDT');
      | set_param([gcb '/SUB'],'IpDT',DTStr);
      | 
      | FColor = '[0.901961, 0.313725, 0.078431]'; 
      | try
      |     set_param([gcb '/y'],'ForegroundColor',FColor);
      |     set_param(gcb,'ForegroundColor',FColor);
      | catch
      | end
      mask Display:
      | % color('red');
      | % disp (sprintf('Hysterisis\nR-Dlt'));
      | image(imread('HysRDlt.jpg'),[0.2,0.1,0.65,0.9]);
  Hysterisis : Subsystem  TreatAsAtomicUnit=on
      mask help: Inputs DV, RV, u, Rst and RstV should have same Data Types, double, single or interger. Rst, RstV and output y are boolean.
      mask init:
      | FColor = '[0.901961, 0.313725, 0.078431]'; 
      | try
      |     set_param([gcb '/y'],'ForegroundColor',FColor);
      |     set_param(gcb,'ForegroundColor',FColor);
      | catch
      | end
      mask Display:
      | % color('red');
      | % disp('\bfHysterisis','texmode','on');
      | image(imread('Hysterisis.jpg'),[0.3,0.15,0.6,0.8]);
  Hysterisis_NoRst : Subsystem  TreatAsAtomicUnit=on
      mask init:
      | FColor = '[0.901961, 0.313725, 0.078431]'; 
      | try
      |     set_param([gcb '/y'],'ForegroundColor',FColor);
      |     set_param(gcb,'ForegroundColor',FColor);
      | catch
      | end
      mask Display: image(imread('Hysterisis.jpg'),[0.3,0.15,0.6,0.8]);
  LIMIT : Subsystem  TreatAsAtomicUnit=on  mask{IpDT=double}
      mask prompts: IpDT "Input Data Type (u, MN and MX)"
      mask help: Dynamic Saturation
      mask init:
      | DTStry = get_param(gcb,'IpDT');
      | try
      |     if isequal(DTStry,'boolean')
      |         FColor = '[0.901961, 0.313725, 0.078431]'; 
      |     elseif isequal(DTStry,'double')||isequal(DTStry,'single')
      |         FColor = '[0.313725, 0.117647, 0.352941]';  
      |     else
      |         FColor = '[0.196078, 0.549020, 0.549020]';
      |     end        
      | catch
      | end
      | set_param([gcb '/y'],'ForegroundColor',FColor);
      | set_param(gcb,'ForegroundColor',FColor);
      | 
      | FColorFlg = '[0.901961, 0.313725, 0.078431]'; 
      | try
      |     set_param([gcb '/MX_Flg'],'ForegroundColor',FColorFlg);
      |     set_param([gcb '/MN_Flg'],'ForegroundColor',FColorFlg);
      | catch
      | end
      mask Display:
      | % color('red');
      | % disp (sprintf('Dynamic\nSaturation'));
      | image(imread('LIMIT.jpg'),[0.2,0.15,0.48,0.8]);
  SIGN : Subsystem  TreatAsAtomicUnit=on  mask{OpDT=double}
      mask prompts: OpDT "Output Data Type"
      mask help: For real input, output 1 for positive input, -1 for negative input, and 0 for 0 input.
      mask init:
      | DTStry = get_param(gcb,'OpDT');
      | try
      |     if isequal(DTStry,'boolean')
      |         FColor = '[0.901961, 0.313725, 0.078431]'; 
      |     elseif isequal(DTStry,'double')||isequal(DTStry,'single')
      |         FColor = '[0.313725, 0.117647, 0.352941]';  
      |     else
      |         FColor = '[0.196078, 0.549020, 0.549020]';
      |     end        
      | catch
      | end
      | set_param([gcb '/y'],'ForegroundColor',FColor);
      | set_param(gcb,'ForegroundColor',FColor);
      mask Display:
      | % disp('Sign');
      | image(imread('SIGN.jpg'),[0.1,0.15,0.95,0.9]);
